simulink model "Sim_PD_XY"  (R2016a)
settings: Solver=VariableStepAuto  SolverMode=SingleTasking  StartTime=0.0  StopTime=10.0  RelTol=1e-3
undefined symbols (not defined in the file): k_reg, k_s, T_1, T_r
libraries: simulink x1
settings Model: Creator=Florian  LastModifiedBy=Florian
settings OptimizationCC: DefaultParameterBehavior=Inlined  UseDivisionForNetSlopeComputation=on  UseFloatMulNetSlope=on  InlineInvariantSignals=on  PassReuseOutputArgsAs=Individual arguments  ZeroExternalMemoryAtStartup=off  ZeroInternalMemoryAtStartup=off  NoFixptDivByZeroProtection=on  EfficientFloat2IntCast=on  OptimizeModelRefInitCode=on  LifeSpan=1
settings HardwareCC: ProdBitPerPointer=32  ProdLargestAtomicInteger=Long  ProdLargestAtomicFloat=Double  ProdWordSize=32  ProdHWDeviceType=ARM Compatible->ARM Cortex
settings RTWCC: SystemTargetFile=ert.tlc  TemplateMakefile=ert_default_tmf  GenerateReport=on  IncludeHyperlinkInReport=on  LaunchReport=on  GenerateTraceInfo=on  GenerateTraceReport=on  GenerateTraceReportSl=on  GenerateTraceReportSf=on  GenerateTraceReportEml=on  GenerateCodeMetricsReport=on
settings CodeAppCC: ForceParamTrailComments=on  IgnoreCustomStorageClasses=off  OperatorAnnotations=on  SimulinkDataObjDesc=on  SFDataObjDesc=on  MATLABFcnDesc=on  InsertBlockDesc=on  MATLABSourceComments=on
settings ERTTargetCC: GenerateSampleERTMain=on  IncludeMdlTerminateFcn=off  CombineSignalStateStructs=on  SupportComplex=off  SupportContinuousTime=on  InlinedParameterPlacement=NonHierarchical  ERTCustomFileTemplate=example_file_process.tlc  ERTFilePackagingFormat=CompactWithDataFile

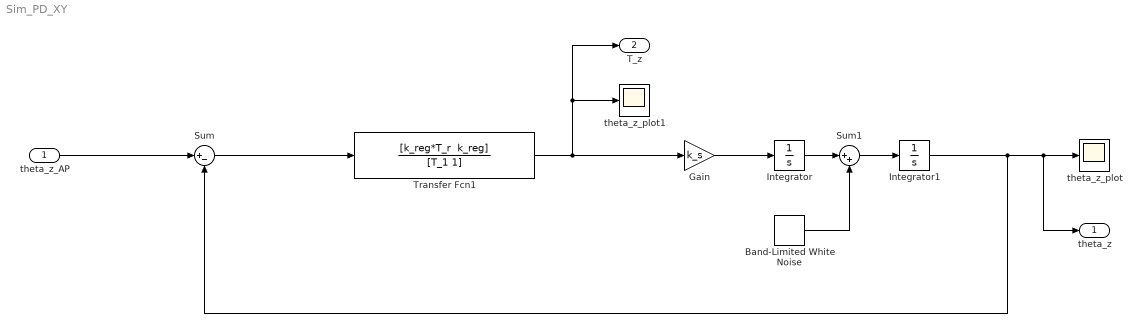
== system Sim_PD_XY ==
  "theta_z_AP " : Inport
  Band-Limited White Noise : simulink/Sources/Band-Limited White Noise  Cov=[0.1^2]  Ts=1/92  seed=[23341]
  Gain : Gain  Gain=k_s
  Integrator : Integrator
  Integrator1 : Integrator  InitialCondition=pi/32
  Sum : Sum  Inputs=|+-
  Sum1 : Sum  Inputs=|++
  Transfer Fcn1 : TransferFcn  Numerator="[k_reg*T_r  k_reg]"  Denominator=[T_1 1]
  theta_z_plot : Scope
  theta_z_plot1 : Scope
  "theta_z " : Outport
  T_z : Outport  Port=2
  wires:
  Sum/1 -> Transfer Fcn1/1
  Gain/1 -> Integrator/1
  Integrator1/1 -> "theta_z "/1, theta_z_plot/1, Sum/2
  "theta_z_AP "/1 -> Sum/1
  Band-Limited White Noise/1 -> Sum1/2
  Integrator/1 -> Sum1/1
  Sum1/1 -> Integrator1/1
  Transfer Fcn1/1 -> Gain/1, T_z/1, theta_z_plot1/1
